simulink model "week1_problem9_2005052"  (R2021a)
settings: Solver=VariableStepAuto  StartTime=0.0  StopTime=120  RelTol=1e-3
model workspace (MAT data in the model file):
  J = 0.01
  K = 0.01
  L = 0.5
  R = 1
  b = 0.1
settings Model: Creator=admin  LastModifiedBy=admin
settings SolverCC: AlgebraicLoopSolver=TrustRegion
settings DebuggingCC: SFMachineParentedDataDiag=warning

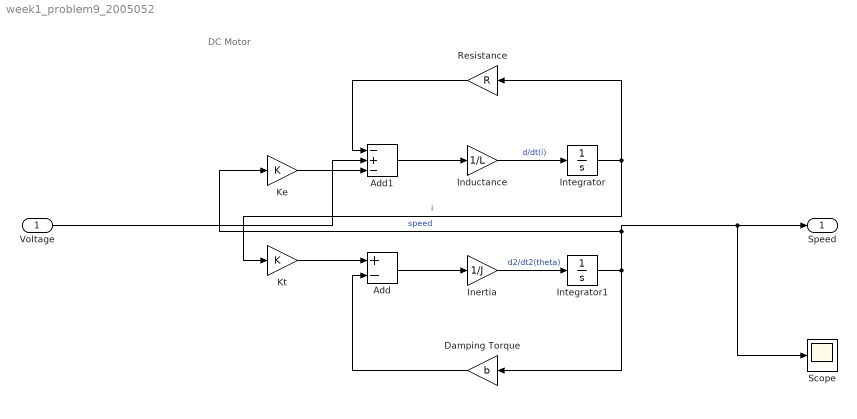
== system week1_problem9_2005052 ==
  note: DC Motor
  Voltage : Inport
  Add : Sum  Inputs=+-
  Add1 : Sum  Inputs=-+-
  Damping Torque : Gain  Gain=b
  Inductance : Gain  Gain=1/L
  Inertia : Gain  Gain=1/J
  Integrator : Integrator
  Integrator1 : Integrator
  Ke : Gain  Gain=K
  Kt : Gain  Gain=K
  Resistance : Gain  Gain=R
  Scope : Scope
  Speed : Outport
  wires:
  Kt/1 -> Add/1
  Damping Torque/1 -> Add/2
  Add/1 -> Inertia/1
  Ke/1 -> Add1/3
  Resistance/1 -> Add1/1
  Inertia/1 -> Integrator1/1  "d2/dt2(theta)"
  Integrator/1 -> Kt/1, Resistance/1  "i"
  Add1/1 -> Inductance/1
  Inductance/1 -> Integrator/1  "d/dt(i)"
  Integrator1/1 -> Scope/1, Speed/1, Ke/1, Damping Torque/1  "speed"
  Voltage/1 -> Add1/2
